simulink model "Punkt_3"  (R2018b)
settings: Solver=VariableStepAuto  StartTime=0.0  StopTime=5  MaxStep=0.01  RelTol=1e-3
InitFcn:
  | GG = [0 1; -9 0];
  | Hg = [1 0];
  | A = [0 1; 4 0];
  | B = [1; 1];
  | Bf = [2; 6];
  | C = [3 0];
  | D = 3;
  | G = [1; 1];
  | 
  | w = 13;
  | syms s;
  | 
  | 
  | GG_ = [0 0 0 -w^4; 1 0 0 -4*w^3; 0 1 0 -6*w^2; 0 0 1 -4*w];
  | H_ = [0 0 0 1];
  | A_ = [GG -G*C; zeros(2) A];
  | B_ = [-G*D; B];
  | 
  | M_ = sylv(-A_, GG_,B_.*H_);
  | K_ = -H_*inv(M_);
  | 
  | Ke = [K_(1) K_(2)];
  | Kx = [K_(3) K_(4)];
  | 
  | Fn = -3
  | Gn = 1;
  | 
  | Mn = sylv(-Fn,A,Gn*C)
  | 
  | N = [C; Mn];
settings Model: Creator=kekos  LastModifiedBy=kekos

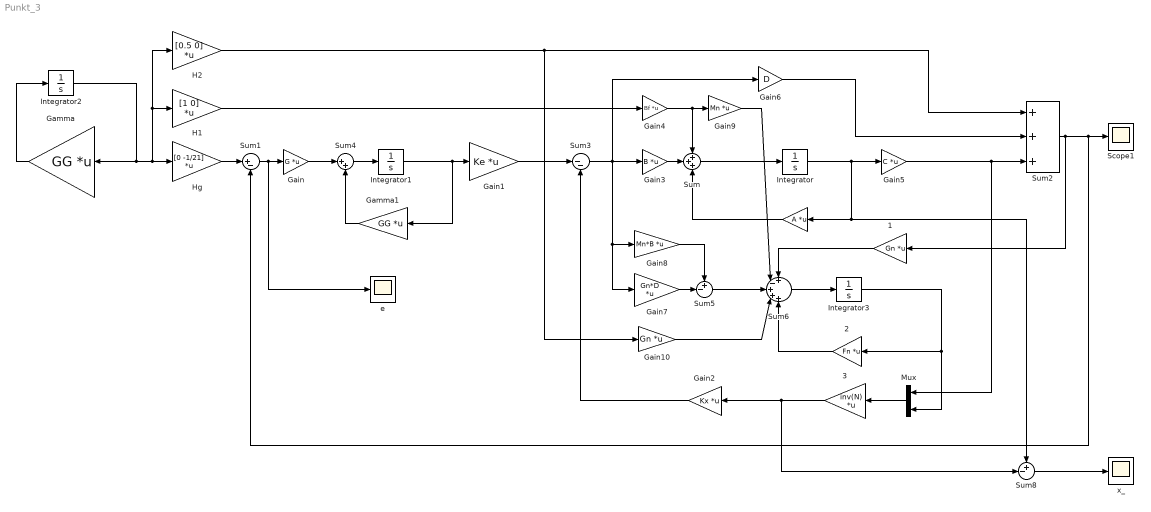
== system Punkt_3 ==
  " " : Gain  Gain=A  Multiplication=Matrix(K*u)
  " 1" : Gain  Gain=Gn  Multiplication=Matrix(K*u)
  " 2" : Gain  Gain=Fn  Multiplication=Matrix(K*u)
  " 3" : Gain  Gain=inv(N)  Multiplication=Matrix(K*u)
  Gain : Gain  Gain=G  Multiplication=Matrix(K*u)
  Gain1 : Gain  Gain=Ke  Multiplication=Matrix(K*u)
  Gain10 : Gain  Gain=Gn  Multiplication=Matrix(K*u)
  Gain2 : Gain  Gain=Kx  Multiplication=Matrix(K*u)
  Gain3 : Gain  Gain=B  Multiplication=Matrix(K*u)
  Gain4 : Gain  Gain=Bf  Multiplication=Matrix(K*u)
  Gain5 : Gain  Gain=C  Multiplication=Matrix(K*u)
  Gain6 : Gain  Gain=D
  Gain7 : Gain  Gain=Gn*D  Multiplication=Matrix(K*u)
  Gain8 : Gain  Gain=Mn*B  Multiplication=Matrix(K*u)
  Gain9 : Gain  Gain=Mn  Multiplication=Matrix(K*u)
  Gamma : Gain  Gain=GG  Multiplication=Matrix(K*u)
  Gamma1 : Gain  Gain=GG  Multiplication=Matrix(K*u)
  H1 : Gain  Gain=[1 0]  Multiplication=Matrix(K*u)
  H2 : Gain  Gain=[0.5 0]  Multiplication=Matrix(K*u)
  Hg : Gain  Gain=[0 -1/21]  Multiplication=Matrix(K*u)
  Integrator : Integrator
  Integrator1 : Integrator  InitialCondition=[-2.91; -19.10]
  Integrator2 : Integrator  InitialCondition=[-2.91; -19.10]
  Integrator3 : Integrator  InitialCondition=1
  Mux : Mux  Inputs=2
  Scope1 : Scope
  Sum : Sum  Inputs=+++
  Sum1 : Sum  Inputs=|+-
  Sum2 : Sum  Inputs=+++
  Sum3 : Sum  Inputs=|--
  Sum4 : Sum  Inputs=|++
  Sum5 : Sum  Inputs=+-|
  Sum6 : Sum  Inputs=+-+++
  Sum8 : Sum  Inputs=+-|
  e : Scope
  x_ : Scope
  wires:
  Sum2/1 -> " 1"/1, Sum1/2, Scope1/1
  H2/1 -> Sum2/1, Gain10/1
  Gamma/1 -> Integrator2/1
  Hg/1 -> Sum1/1
  Sum1/1 -> Gain/1, e/1
  Integrator1/1 -> Gain1/1, Gamma1/1
  Sum4/1 -> Integrator1/1
  Gain/1 -> Sum4/1
  Gamma1/1 -> Sum4/2
  Gain2/1 -> Sum3/2
  Integrator/1 -> Gain5/1, Sum8/1, " "/1
  " "/1 -> Sum/3
  Gain6/1 -> Sum2/2
  Sum3/1 -> Gain8/1, Gain7/1, Gain3/1, Gain6/1
  Sum/1 -> Integrator/1
  H1/1 -> Gain4/1
  Gain4/1 -> Gain9/1, Sum/1
  Gain7/1 -> Sum5/2
  Gain3/1 -> Sum/2
  " 1"/1 -> Sum6/1
  Integrator3/1 -> Mux/2, " 2"/1
  Sum6/1 -> Integrator3/1
  " 3"/1 -> Gain2/1, Sum8/2
  Mux/1 -> " 3"/1
  Sum8/1 -> x_/1
  Gain5/1 -> Mux/1, Sum2/3
  Integrator2/1 -> H2/1, H1/1, Hg/1, Gamma/1
  Gain1/1 -> Sum3/1
  Gain8/1 -> Sum5/1
  " 2"/1 -> Sum6/5
  Sum5/1 -> Sum6/3
  Gain9/1 -> Sum6/2
  Gain10/1 -> Sum6/4
